simulink model "openMHA_test_db_lookup_gain_fpga"  (R2020a)
settings: Solver=VariableStepAuto  StartTime=0.0  StopTime=stop_time  RelTol=1e-3
InitFcn:
  | test_db_lookup_gain_fpga_init
StopFcn:
  | test_db_lookup_gain_fpga_stop
values from neighbouring files (symbols this model uses):
  table_length = length(gtdata)    [calculate_gaintable.m]    (also in test_FFT_to_gain_init.m; test_ar_filter_gaintable_init.m; test_db_ar_gaintable_init.m; test_db_lookup_gain_fpga_init.m)
  X_high = 93    [test_FFT_to_gain_init.m]    (also in test_ar_filter_gaintable_init.m = 95; test_db_ar_gaintable_init.m; test_db_lookup_gain_fpga_init.m = 95; test_db_lookup_init.m = 95)
  xIn = [4.65661287308e-10 5.23868948221e-10 5.82076609135e-10 6.40284270048e-10 6.98491930962e-10 7.56699591875e-10 8.14907252789e-10 8.73114913702e-10 9.31322574615e-10 1.04773789644e-09 1.16415321827e-09 1.2805685401e-09 ... (256 elements, 1x256)]    [openMHA_test_db_lookup_gain_Programmable Look-Up Table_init.mat]    (also in openMHA_test_db_lookup_gain_Programmable Lookup Table dB_init.mat = [4.65661287308e-10 4.72937244922e-10 4.80213202536e-10 4.874)
libraries: FPGA_Open_Speech_Tools x2, dspsrcs4 x1, simulink x1
settings Model: PacingRate=10  Creator=t96f346  LastModifiedBy=t96f346
settings OptimizationCC: BlockReduction=off  ConditionallyExecuteInputs=off  DefaultParameterBehavior=Inlined
settings DebuggingCC: AlgebraicLoopMsg=error
settings HardwareCC: ProdBitPerPointer=32  ProdBitPerSizeT=32  ProdBitPerPtrDiffT=32  ProdLargestAtomicFloat=None  ProdIntDivRoundTo=Undefined  ProdEndianess=Unspecified  ProdWordSize=32  ProdHWDeviceType=ASIC/FPGA->ASIC/FPGA  TargetBitPerPointer=64  TargetBitPerSizeT=64  TargetBitPerPtrDiffT=64  TargetLongLongMode=on  TargetIntDivRoundTo=Zero  TargetEndianess=LittleEndian  TargetWordSize=64  TargetHWDeviceType=Custom Processor->MATLAB Host Computer  ProdEqTarget=off

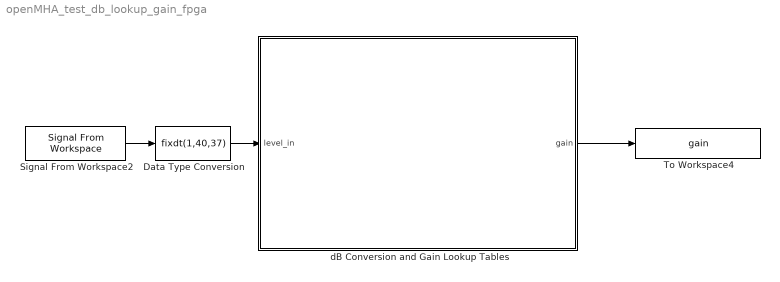
== system openMHA_test_db_lookup_gain_fpga ==
  Data Type Conversion : DataTypeConversion  OutDataTypeStr=fixdt(1,40,37)
  Signal From Workspace2 : dspsrcs4/Signal From Workspace  X=level_in  Ts=1  nsamps=1  OutputAfterFinalValue=Setting to zero  ignoreOrWarnInputAndFrameLengths=off  OutputFrames=off
  To Workspace4 : ToWorkspace  VariableName=gain  SampleTime=-1
      settings: Save2DSignal=2-D array (concatenate along first dimension)
  dB Conversion and Gain Lookup Tables : Subsystem
  wires:
  Signal From Workspace2/1 -> Data Type Conversion/1
  dB Conversion and Gain Lookup Tables/1(gain) -> To Workspace4/1
  Data Type Conversion/1 -> dB Conversion and Gain Lookup Tables/1(level_in)

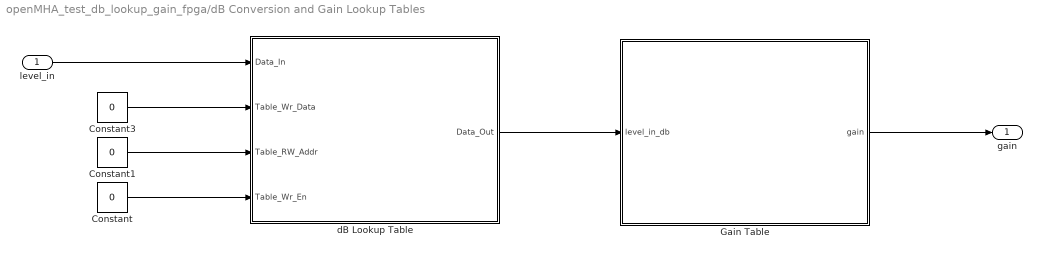
== system openMHA_test_db_lookup_gain_fpga/dB Conversion and Gain Lookup Tables ==
  level_in : Inport
  Constant : Constant  Value=0  OutDataTypeStr=boolean  SampleTime=-1
  Constant1 : Constant  Value=0  OutDataTypeStr=uint16  SampleTime=-1
  Constant3 : Constant  Value=0  OutDataTypeStr=fixdt(1,40,32)  SampleTime=-1
  Gain Table : Subsystem
  dB Lookup Table : Subsystem
  gain : Outport
  wires:
  Constant/1 -> dB Lookup Table/4(Table_Wr_En)
  dB Lookup Table/1(Data_Out) -> Gain Table/1(level_in_db)
  Constant1/1 -> dB Lookup Table/3(Table_RW_Addr)
  level_in/1 -> dB Lookup Table/1(Data_In)
  Constant3/1 -> dB Lookup Table/2(Table_Wr_Data)
  Gain Table/1(gain) -> gain/1

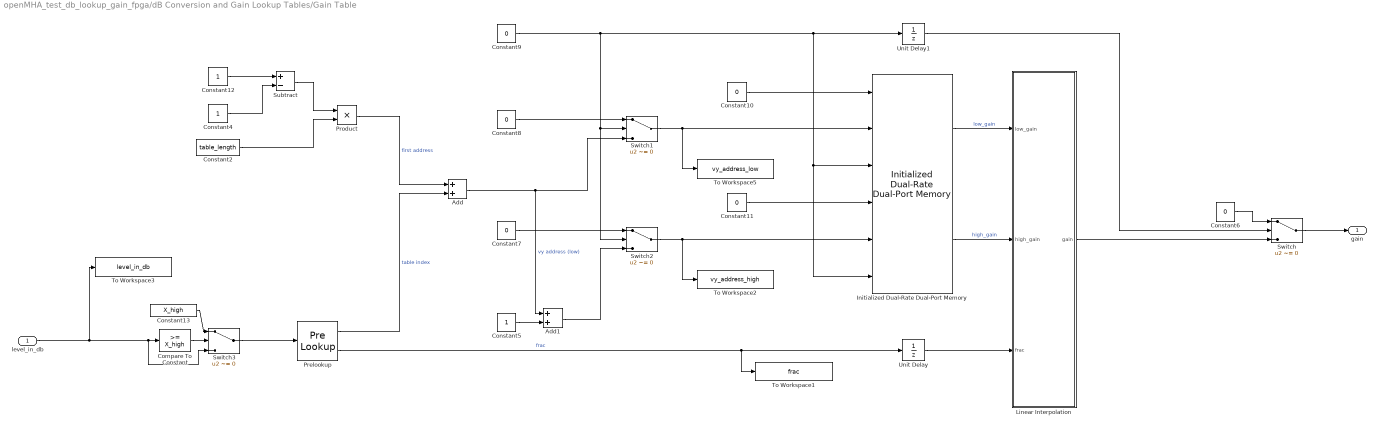
== system openMHA_test_db_lookup_gain_fpga/dB Conversion and Gain Lookup Tables/Gain Table ==
  level_in_db : Inport
  Add : Sum  OutDataTypeStr=uint8
  Add1 : Sum  OutDataTypeStr=uint8
  Compare To Constant : simulink/Logic and Bit Operations/Compare To Constant  relop=>=  const=X_high  OutDataTypeStr=boolean
  Constant10 : Constant  Value=0  OutDataTypeStr=fixdt(1,16,8)  SampleTime=-1
  Constant11 : Constant  Value=0  OutDataTypeStr=fixdt(1,16,8)  SampleTime=-1
  Constant12 : Constant  OutDataTypeStr=uint8  SampleTime=-1
  Constant13 : Constant  Value=X_high  OutDataTypeStr=fixdt(1,Wbits, Fbits-5)  SampleTime=-1
  Constant2 : Constant  Value=table_length  OutDataTypeStr=uint8  SampleTime=-1
  Constant4 : Constant  OutDataTypeStr=uint8  SampleTime=-1
  Constant5 : Constant  OutDataTypeStr=uint8  SampleTime=-1
  Constant6 : Constant  Value=0  OutDataTypeStr=fixdt(1,16,8)  SampleTime=-1
  Constant7 : Constant  Value=0  OutDataTypeStr=uint8  SampleTime=-1
  Constant8 : Constant  Value=0  OutDataTypeStr=uint8  SampleTime=-1
  Constant9 : Constant  Value=0  OutDataTypeStr=boolean  SampleTime=-1
  Initialized Dual-Rate Dual-Port Memory : FPGA_Open_Speech_Tools/Initialized Dual-Rate Dual-Port Memory  ram_size=RAM_size  Table_Init=vy
      settings: SourceProductName=FPGA Open Speech Tools
  Linear Interpolation : Subsystem
  Prelookup : PreLookup  BreakpointsData=input_levels_db  IndexSearchMethod=Evenly spaced points  UseLastBreakpoint=on  DiagnosticForOutOfRangeInput=Error  IndexDataTypeStr=uint8
  Product : Product  OutDataTypeStr=Inherit: Same as first input
  Subtract : Sum  Inputs=+-
  Switch : Switch  Criteria=u2 ~= 0
  Switch1 : Switch  Criteria=u2 ~= 0  OutDataTypeStr=uint8
  Switch2 : Switch  Criteria=u2 ~= 0  OutDataTypeStr=uint8
  Switch3 : Switch  Criteria=u2 ~= 0
  To Workspace1 : ToWorkspace  VariableName=frac  SampleTime=-1
      settings: Save2DSignal=2-D array (concatenate along first dimension)
  To Workspace2 : ToWorkspace  VariableName=vy_address_high  SampleTime=-1
      settings: Save2DSignal=2-D array (concatenate along first dimension)
  To Workspace3 : ToWorkspace  VariableName=level_in_db  SampleTime=-1
      settings: Save2DSignal=2-D array (concatenate along first dimension)
  To Workspace5 : ToWorkspace  VariableName=vy_address_low  SampleTime=-1
      settings: Save2DSignal=2-D array (concatenate along first dimension)
  Unit Delay : UnitDelay  SampleTime=-1  HasFrameUpgradeWarning=on
  Unit Delay1 : UnitDelay  InitialCondition=1  SampleTime=-1  HasFrameUpgradeWarning=on
  gain : Outport
  wires:
  Constant9/1 -> Initialized Dual-Rate Dual-Port Memory/3, Initialized Dual-Rate Dual-Port Memory/6, Unit Delay1/1, Switch1/2, Switch2/2
  Initialized Dual-Rate Dual-Port Memory/1 -> Linear Interpolation/1(low_gain)  "low_gain"
  Switch2/1 -> Initialized Dual-Rate Dual-Port Memory/5, To Workspace2/1
  Constant11/1 -> Initialized Dual-Rate Dual-Port Memory/4
  Constant12/1 -> Subtract/1
  Subtract/1 -> Product/1
  Add1/1 -> Switch2/3
  Product/1 -> Add/1  "first address"
  Prelookup/1 -> Add/2  "table index"
  Prelookup/2 -> To Workspace1/1, Unit Delay/1  "frac"
  Linear Interpolation/1(gain) -> Switch/3
  Switch1/1 -> Initialized Dual-Rate Dual-Port Memory/2, To Workspace5/1
  Initialized Dual-Rate Dual-Port Memory/2 -> Linear Interpolation/2(high_gain)  "high_gain"
  Constant7/1 -> Switch2/1
  level_in_db/1 -> To Workspace3/1, Switch3/3, Compare To Constant/1
  Compare To Constant/1 -> Switch3/2
  Constant13/1 -> Switch3/1
  Constant10/1 -> Initialized Dual-Rate Dual-Port Memory/1
  Constant6/1 -> Switch/1
  Unit Delay/1 -> Linear Interpolation/3(frac)
  Switch3/1 -> Prelookup/1
  Constant5/1 -> Add1/2
  Unit Delay1/1 -> Switch/2
  Constant8/1 -> Switch1/1
  Add/1 -> Switch1/3, Add1/1  "vy address (low)"
  Constant4/1 -> Subtract/2
  Constant2/1 -> Product/2
  Switch/1 -> gain/1

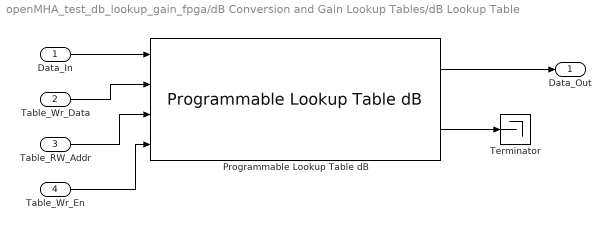
== system openMHA_test_db_lookup_gain_fpga/dB Conversion and Gain Lookup Tables/dB Lookup Table ==
  Data_In : Inport
  Table_Wr_Data : Inport  Port=2
  Table_RW_Addr : Inport  Port=3
  Table_Wr_En : Inport  Port=4
  Programmable Lookup Table dB : FPGA_Open_Speech_Tools/Programmable Lookup Table dB  tableFnParam=10.*log10(2500000000.*xIn)  SAVE_TABLE=off  maxInput=1  floorParam=2^-31  errorParam=1  ERR_DIAG=on  PLOT_TABLE=off  nBitsParam=5  mBitsParam=4  IGOTTHIS=off  W_bits=40  F_bits=37  tableInit=0  binaryOffset=0
      settings: SourceProductName=FPGA Open Speech Tools
  Terminator : Terminator
  Data_Out : Outport
  wires:
  Programmable Lookup Table dB/2 -> Terminator/1
  Data_In/1 -> Programmable Lookup Table dB/1
  Programmable Lookup Table dB/1 -> Data_Out/1
  Table_Wr_En/1 -> Programmable Lookup Table dB/4
  Table_Wr_Data/1 -> Programmable Lookup Table dB/2
  Table_RW_Addr/1 -> Programmable Lookup Table dB/3

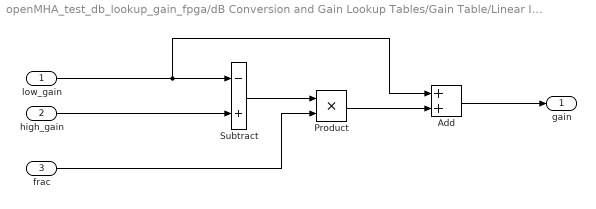
== system openMHA_test_db_lookup_gain_fpga/dB Conversion and Gain Lookup Tables/Gain Table/Linear Interpolation ==
  low_gain : Inport
  high_gain : Inport  Port=2
  frac : Inport  Port=3
  Add : Sum
  Product : Product  OutDataTypeStr=Inherit: Same as first input
  Subtract : Sum  Inputs=-+
  gain : Outport
  wires:
  high_gain/1 -> Subtract/2
  low_gain/1 -> Add/1, Subtract/1
  Subtract/1 -> Product/1
  frac/1 -> Product/2
  Product/1 -> Add/2
  Add/1 -> gain/1
